simulink model "drone2"  (R2022a)
settings: Solver=FixedStepAuto  StartTime=0.0  StopTime=10.0  FixedStep=1  RelTol=1e-3
settings Model: Creator=JadKHaddad  LastModifiedBy=JadKHaddad

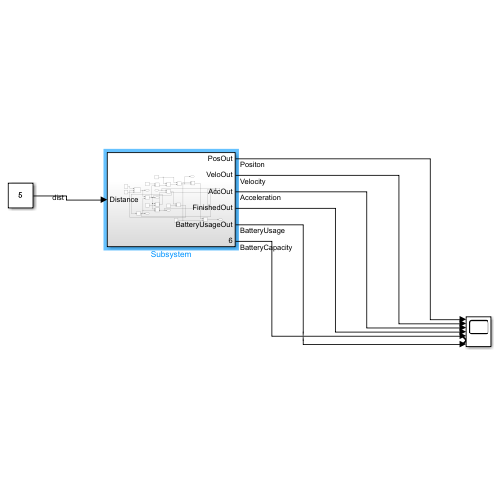
[thumbnail: Simulink's stored preview of the top-level diagram]
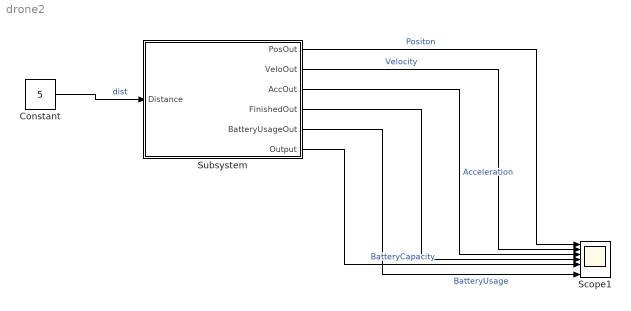
== system drone2 ==
  Constant : Constant  Value=5
  Scope1 : Scope  NumInputPorts=7
  Subsystem : Subsystem
  wires:
  Constant/1 -> Subsystem/1(Distance)  "dist"
  Subsystem/3(AccOut) -> Scope1/3  "Acceleration"
  Subsystem/5(BatteryUsageOut) -> Scope1/7  "BatteryUsage"
  Subsystem/1(PosOut) -> Scope1/1  "Positon"
  Subsystem/4(FinishedOut) -> Scope1/4
  Subsystem/6(Output) -> Scope1/5  "BatteryCapacity"
  Subsystem/2(VeloOut) -> Scope1/2  "Velocity"

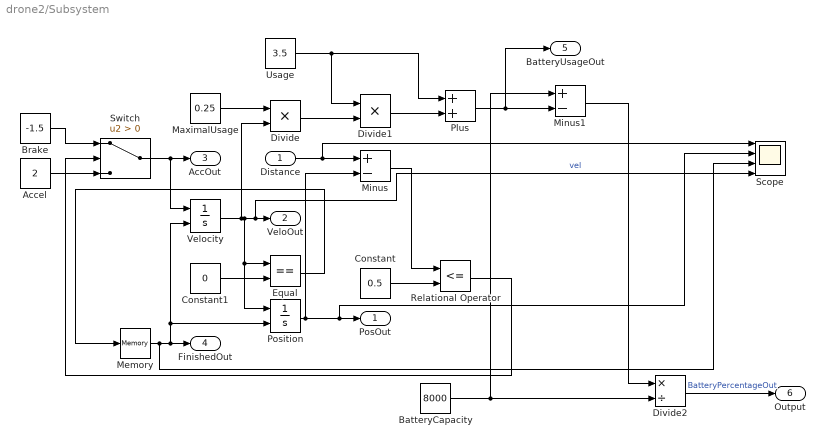
== system drone2/Subsystem ==
  Distance : Inport
  Accel : Constant  Value=2
  BatteryCapacity : Constant  Value=8000
  Brake : Constant  Value=-1.5
  Constant : Constant  Value=0.5
  Constant1 : Constant  Value=0
  Divide : Product  Inputs=**  RndMeth=Round
  Divide1 : Product  Inputs=**
  Divide2 : Product  Inputs=*/
  Equal : RelationalOperator  Operator===  OutDataTypeStr=boolean  RndMeth=Simplest  InputSameDT=off
  MaximalUsage : Constant  Value=0.25
  Memory : Memory
  Minus : Sum  Inputs=+-
  Minus1 : Sum  Inputs=+-
  Plus : Sum
  Position : Integrator  ExternalReset=rising
  Relational Operator : RelationalOperator  Operator=<=  OutDataTypeStr=boolean  RndMeth=Simplest  InputSameDT=off
  Scope : Scope  NumInputPorts=4
  Switch : Switch  Criteria=u2 > Threshold  SaturateOnIntegerOverflow=off  InputSameDT=off
  Usage : Constant  Value=3.5
  Velocity : Integrator  ExternalReset=rising  LimitOutput=on  UpperSaturationLimit=1  LowerSaturationLimit=0
  PosOut : Outport
  VeloOut : Outport  Port=2
  AccOut : Outport  Port=3
  FinishedOut : Outport  Port=4
  BatteryUsageOut : Outport  Port=5
  Output : Outport  Port=6
  wires:
  Position/1 -> Minus/2, Scope/2, PosOut/1
  Relational Operator/1 -> Switch/2
  Minus1/1 -> Divide2/1
  Divide2/1 -> Output/1  "BatteryPercentageOut"
  MaximalUsage/1 -> Divide/1
  Divide/1 -> Divide1/2
  Divide1/1 -> Plus/2
  Memory/1 -> Scope/3, Velocity/2, Position/2, FinishedOut/1
  Distance/1 -> Scope/1, Minus/1
  Constant/1 -> Relational Operator/2
  Constant1/1 -> Equal/2
  Brake/1 -> Switch/1
  Equal/1 -> Memory/1
  Minus/1 -> Relational Operator/1
  Switch/1 -> Velocity/1, AccOut/1
  Accel/1 -> Switch/3
  BatteryCapacity/1 -> Minus1/1, Divide2/2
  Usage/1 -> Plus/1, Divide1/1
  Velocity/1 -> Equal/1, Position/1, Scope/4, VeloOut/1, Divide/2  "vel"
  Plus/1 -> Minus1/2, BatteryUsageOut/1
